simulink model "DC_Motor1"  (R2019b)
settings: Solver=VariableStepAuto  StartTime=0.0  StopTime=10.0  RelTol=1e-3
values from neighbouring files (symbols this model uses):
  Beq = 0.015    [DC_Motor.m]
  Ith = 1.6*Imax    (= 1.6)    [DC_Motor.m]
  Jeq = 2.087e-3    (= 0.002087)    [DC_Motor.m]
  Km = 7.68e-3    (= 0.00768)    [DC_Motor.m]
  Kp_i = Wci*Lm    (= 2.6)    [DC_Motor.m]
  Kp_p = Wcp    (= 0.718735026354)    [DC_Motor.m]
  Kp_v = Wcv*Jeq    (= 0.015)    [DC_Motor.m]
  Kt = 7.68e-3    (= 0.00768)    [DC_Motor.m]
  Lm = 0.18e-3    (= 0.00018)    [DC_Motor.m]
  Rm = 2.6    [DC_Motor.m]
  Ti_i = Kp_i/Ki_i    (= 6.92307692308e-05)    [DC_Motor.m]
  Ti_v = Kp_v/Ki_v    (= 0.139133333333)    [DC_Motor.m]
  Vth = 1*Vnom    (= 6)    [DC_Motor.m]
settings Model: Creator=francescomarata  LastModifiedBy=francescomarata

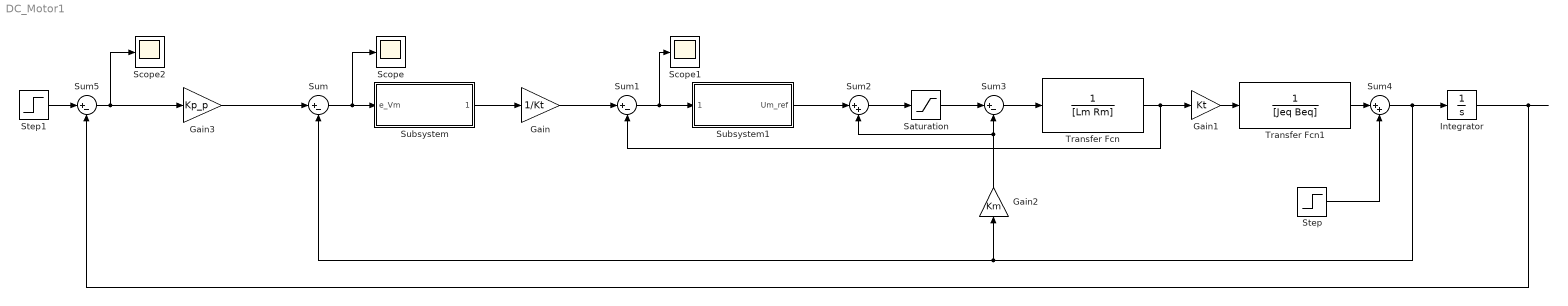
== system DC_Motor1 ==
  Gain : Gain  Gain=1/Kt
  Gain1 : Gain  Gain=Kt
  Gain2 : Gain  Gain=Km
  Gain3 : Gain  Gain=Kp_p
  Integrator : Integrator
  Saturation : Saturate  UpperLimit=Vth  LowerLimit=-Vth
  Scope : Scope
  Scope1 : Scope
  Scope2 : Scope
  Step : Step  Time=3  After=0.3  SampleTime=0
  Step1 : Step  Time=0  After=pi/2  SampleTime=0
  Subsystem : Subsystem
  Subsystem1 : Subsystem
  Sum{,1,3,5} (4 alike) : Sum  Inputs=|+-
  Sum2 : Sum  Inputs=|++
  Sum4 : Sum  Inputs=|++
  Transfer Fcn : TransferFcn  Denominator=[Lm Rm]
  Transfer Fcn1 : TransferFcn  Denominator=[Jeq Beq]
  wires:
  Transfer Fcn/1 -> Sum1/2, Gain1/1
  Sum3/1 -> Transfer Fcn/1
  Gain/1 -> Sum1/1
  Gain1/1 -> Transfer Fcn1/1
  Sum2/1 -> Saturation/1
  Saturation/1 -> Sum3/1
  Gain2/1 -> Sum2/2, Sum3/2
  Sum1/1 -> Scope1/1, Subsystem1/1(" ")
  Subsystem1/1("Um_ref ") -> Sum2/1
  Subsystem/1(" ") -> Gain/1
  Sum/1 -> Scope/1, Subsystem/1("e_Vm ")
  Transfer Fcn1/1 -> Sum4/1
  Sum4/1 -> Integrator/1, Gain2/1, Sum/2
  Step/1 -> Sum4/2
  Integrator/1 -> Sum5/2
  Step1/1 -> Sum5/1
  Sum5/1 -> Scope2/1, Gain3/1
  Gain3/1 -> Sum/1

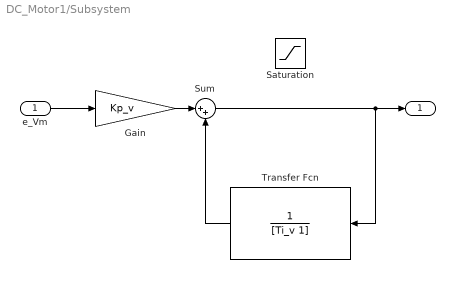
== system DC_Motor1/Subsystem ==
  "e_Vm " : Inport
  Gain : Gain  Gain=Kp_v
  Saturation : Saturate  UpperLimit=Ith  LowerLimit=-Ith
  Sum : Sum  Inputs=|++
  Transfer Fcn : TransferFcn  Denominator=[Ti_v 1]
  " " : Outport
  wires:
  "e_Vm "/1 -> Gain/1
  Gain/1 -> Sum/1
  Transfer Fcn/1 -> Sum/2
  Sum/1 -> Transfer Fcn/1, " "/1

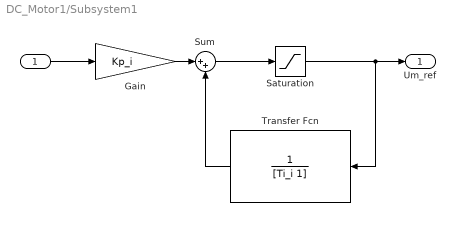
== system DC_Motor1/Subsystem1 ==
  " " : Inport
  Gain : Gain  Gain=Kp_i
  Saturation : Saturate  UpperLimit=Vth  LowerLimit=-Vth
  Sum : Sum  Inputs=|++
  Transfer Fcn : TransferFcn  Denominator=[Ti_i 1]
  "Um_ref " : Outport
  wires:
  Transfer Fcn/1 -> Sum/2
  Sum/1 -> Saturation/1
  " "/1 -> Gain/1
  Saturation/1 -> Transfer Fcn/1, "Um_ref "/1
  Gain/1 -> Sum/1
